simulink model "primes"  (Simulink 6.1)
settings: Solver=FixedStepDiscrete  StartTime=0.0  StopTime=5000  RelTol=1e-3
libraries: simulink x3
settings Model: Creator=campa  LastModifiedBy=gcampa
settings DataIOCC: SaveOutput=off  SignalLogging=off  SaveTime=off
settings OptimizationCC: InlineInvariantSignals=off  InitFltsAndDblsToZero=off
settings DebuggingCC: SignalResolutionControl=UseLocalSettings  SolverPrmCheckMsg=warning  MultiTaskDSMMsg=error
settings HardwareCC: TargetHWDeviceType=32-bit Generic

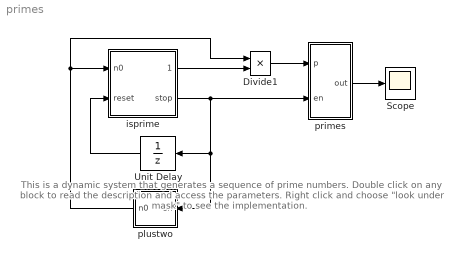
== system primes ==
  note: This is a dynamic system that generates
      | a sequence of prime numbers.
      |
      | Double click on any block to read the
      | description and access the parameters.
      | Right click and choose "look under mask"
      | to see the implementation.
  Divide1 : Product  Inputs=**  OutDataType=fixdt(1,16,0)  OutScaling=[]
  Scope : Scope
      settings: TimeRange=5000  YMin=0  YMax=200  SaveName=p7m  DataFormat=Array
  Unit Delay : UnitDelay  Orientation=left
  isprime : Subsystem  mask(Is Prime){T=1}
      mask prompts: T "Sample Time"
      mask help:
      | This block takes two inputs, the first is a positive number n0 and the second is a reset condition. When the reset input is one, then the block resets its internal state to n0, and it starts dividing n0 for decreasing numbers, until either a factor is found or n0 is found to be prime.
      |
      | When either of the two conditions is met, then the stop output is set to 1, and the isprime output indicates whether n0 is prime or not. Note that if stop==0, then a decision about the primeness of n0 has not been reached yet, and the value of the isprime output is not (yet) significant.
      |
      | The equations of this block are essentially equivalent to the following ones:
      | x(t+1) =  x(t)-sgn(mod(n0,x(t)-1))*sgn(x(t)-3)
      | y(t)     =  sgn(mod(n0,x(t)-1))
      | where sgn(x)=ceil(x/(abs(x)+eps)) is the sign function,  (that is +1 for x>0,  0 for x=0, and -1 for x<0) and n0 is prime when y(inf)=1, while it is not prime when y(inf)==0
      mask Help:
      | This block takes two inputs, the first is a positive number n0 and the second is a reset condition. When the reset input is one, then the block resets its internal state to n0, and it starts dividing n0 for decreasing numbers, until either a factor is found or n0 is found to be prime.
      | <p>
      | When either of the two conditions is met, then the stop output is set to 1, and the isprime output indicates whether n0 is prime or not. Note that if stop==0, then a decision about the primeness of n0 has not been reached yet, and the value of the isprime output is not (yet) significant.
      | <p>
      | The equations of this block are essentially equivalent to the following ones: <br>
      | x(t+1) = x(t)-sgn(mod(n0,x(t)-1))*sgn(x(t)-3) <br>
      | y(t)     = sgn(mod(n0,x(t)-1)) <br>
      | where sgn(x)=ceil(x/(abs(x)+eps)) is the sign function,  (that is +1 for x more than 0,  0 for x=0, and -1 for x less than 0) and n0 is prime when y(inf)=1, while it is not prime when y(inf)==0
  plustwo : Subsystem  Orientation=left  mask(Plus Two){T=1}
      mask prompts: T "Sample Time"
      mask help: Whenever this block is executed (at each sample time), the output is incremented by 2 whenever the input is above 0.5. Otherwise, the optput is kept contsant.
      mask Help: Whenever this block is executed (at each sample time), the output is incremented by 2 whenever the input is above 0.5. Otherwise, the optput is kept constant.
  primes : Subsystem  mask(Primes){T=1}
      mask prompts: T "Sample Time"
      mask help: At each sample time, the first input passes through whenever the second input is above 0.5. Otherwise, the optput is kept constant.
      mask Help: At each sample time, the first input passes through whenever the second input is above 0.5. Otherwise, the optput is kept constant.
  wires:
  isprime/2(stop) -> primes/2(en), plustwo/1(en), Unit Delay/1
  Unit Delay/1 -> isprime/2(reset)
  Divide1/1 -> primes/1(p)
  plustwo/1(n0) -> isprime/1(n0), Divide1/1
  isprime/1(isprime) -> Divide1/2
  primes/1(out) -> Scope/1

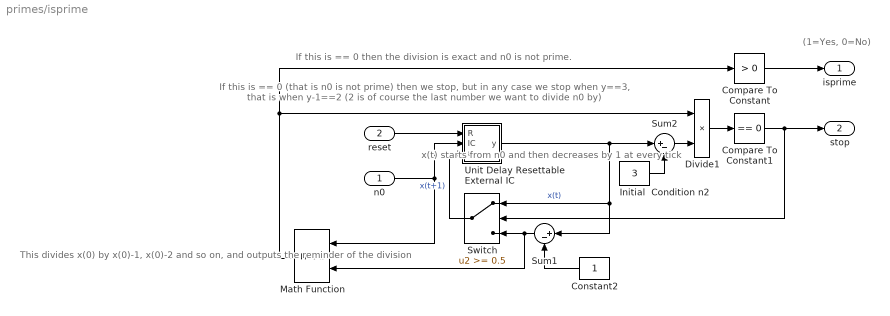
== system primes/isprime ==
  note: If this is == 0 then the division is exact and n0 is not prime.
  note: If this is == 0 (that is n0 is not prime) then we stop,
      | but in any case we stop when y==3, that is when y-1==2
      | (2 is of course the last number we want to divide n0 by)
  note: This divides x(0)
      | by x(0)-1, x(0)-2
      | and so on, and outputs
      | the reminder of the division
  note: x(t) starts from n0
      | and then decreases
      | by 1 at every tick
  note: (1=Yes, 0=No)
  n0 : Inport  Port=1  OutDataType=fixdt(1,16,0)  OutScaling=[]  LatchInput=off
  reset : Inport  Port=2  OutDataType=fixdt(1,16,0)  OutScaling=[]  LatchInput=off
  Compare To Constant : simulink/Logic and Bit Operations/Compare To Constant  relop=>  const=0  LogicOutDataTypeMode=uint8
  Compare To Constant1 : simulink/Logic and Bit Operations/Compare To Constant  relop===  const=0  LogicOutDataTypeMode=boolean
  Constant2 : Constant  Orientation=left  OutDataType=fixdt(1,16,0)  OutScaling=[]
  Divide1 : Product  Inputs=**  OutDataType=fixdt(1,16,0)  OutScaling=[]
  Initial  Condition n2 : Constant  Value=3  OutDataType=fixdt(1,16,0)  OutScaling=[]
  Math Function : Math  Orientation=left  Operator=mod  OutDataType=fixdt(1,16,0)  OutScaling=[]  SaturateOnIntegerOverflow=on
  Sum1 : Sum  Orientation=left  Inputs=|+-  OutDataType=fixdt(1,16,0)  OutScaling=[]
  Sum2 : Sum  Inputs=|+-  OutDataType=fixdt(1,16,0)  OutScaling=[]
  Switch : Switch  Orientation=left  Threshold=0.5
  Unit Delay Resettable External IC : Subsystem  mask(Unit Delay Resettable External Initial Condition){tsamp=T}
      mask prompts: tsamp "Sample time:"
      mask help:
      | Normally, the output is the signal u delayed by one sample period.
      | When the reset signal R is true, the state and the output are always set equal to the initial condition signal IC.  This reset action is vectorized and supports scalar expansion.
      mask Display: dpoly(1,[1 0],'z')
  isprime : Outport  OutDataType=fixdt(1,16,0)  OutScaling=[]
  stop : Outport  Port=2  OutDataType=fixdt(1,16,0)  OutScaling=[]
  wires:
  Constant2/1 -> Sum1/2
  Unit Delay Resettable External IC/1(y) -> Sum2/1, Switch/1, Sum1/1  "x(t)"
  Sum1/1 -> Math Function/2, Switch/3
  n0/1 -> Unit Delay Resettable External IC/2(IC), Math Function/1
  Initial  Condition n2/1 -> Sum2/2
  Math Function/1 -> Divide1/1, Compare To Constant/1
  Sum2/1 -> Divide1/2
  Divide1/1 -> Compare To Constant1/1
  Compare To Constant/1 -> isprime/1
  Compare To Constant1/1 -> stop/1, Switch/2
  reset/1 -> Unit Delay Resettable External IC/1(R)
  Switch/1 -> Unit Delay Resettable External IC/3(u)  "x(t+1)"

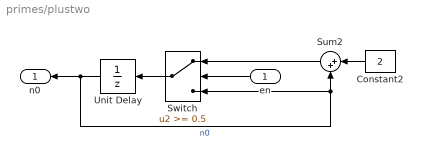
== system primes/plustwo ==
  en : Inport  Orientation=left  Port=1  LatchInput=off
  Constant2 : Constant  Orientation=left  Value=2  OutDataType=fixdt(1,16,0)  OutScaling=[]
  Sum2 : Sum  Orientation=left  Inputs=|++  OutDataType=fixdt(1,16,0)  OutScaling=[]
  Switch : Switch  Orientation=left  Threshold=0.5  SampleTime=T
  Unit Delay : UnitDelay  Orientation=left  X0=3  SampleTime=T
  n0 : Outport  Orientation=left
  wires:
  Switch/1 -> Unit Delay/1
  Sum2/1 -> Switch/1
  Unit Delay/1 -> Sum2/2, Switch/3, n0/1  "n0"
  Constant2/1 -> Sum2/1
  en/1 -> Switch/2

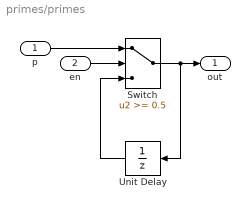
== system primes/primes ==
  p : Inport  Port=1  LatchInput=off
  en : Inport  Port=2  LatchInput=off
  Switch : Switch  Threshold=0.5  SampleTime=T
  Unit Delay : UnitDelay  Orientation=left  SampleTime=T
  out : Outport
  wires:
  Switch/1 -> Unit Delay/1, out/1
  Unit Delay/1 -> Switch/3
  en/1 -> Switch/2
  p/1 -> Switch/1

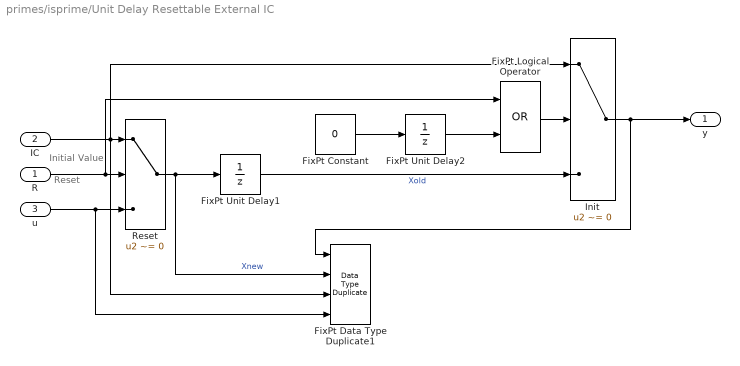
== system primes/isprime/Unit Delay Resettable External IC ==
  note: Reset
  note: Initial Value
  R : Inport  Port=1  OutDataType=fixdt(1,16,0)  OutScaling=[]  LatchInput=off
  IC : Inport  Port=2  OutDataType=fixdt(1,16,0)  OutScaling=[]  LatchInput=off
  u : Inport  Port=3  OutDataType=fixdt(1,16,0)  OutScaling=[]  LatchInput=off
  FixPt Constant : Constant  DisableCoverage=on  Value=0  OutDataType=fixdt(1,16,0)  OutScaling=[]
  FixPt Data Type Duplicate1 : simulink/Signal Attributes/Data Type Duplicate  NumInputPorts=4
  FixPt Logical Operator : Logic  DisableCoverage=on  Operator=OR  AllPortsSameDT=off
  FixPt Unit Delay1 : UnitDelay  DisableCoverage=on  X0=0.0  SampleTime=tsamp
  FixPt Unit Delay2 : UnitDelay  DisableCoverage=on  X0=1  SampleTime=tsamp
  Init : Switch  Criteria=u2 ~= 0  ZeroCross=off
  Reset : Switch  Criteria=u2 ~= 0  ZeroCross=off
  y : Outport  OutDataType=fixdt(1,16,0)  OutScaling=[]
  wires:
  FixPt Logical Operator/1 -> Init/2
  FixPt Unit Delay1/1 -> Init/3  "Xold"
  Init/1 -> y/1, FixPt Data Type Duplicate1/1
  FixPt Unit Delay2/1 -> FixPt Logical Operator/2
  FixPt Constant/1 -> FixPt Unit Delay2/1
  R/1 -> FixPt Logical Operator/1, Reset/2
  Reset/1 -> FixPt Unit Delay1/1, FixPt Data Type Duplicate1/2  "Xnew"
  u/1 -> Reset/3, FixPt Data Type Duplicate1/4
  IC/1 -> FixPt Data Type Duplicate1/3, Init/1, Reset/1
